simulink model "primary_node"  (Simulink 7.8)
settings: Solver=FixedStepDiscrete  SolverMode=SingleTasking  StartTime=0.0  StopTime=10.0  FixedStep=0.01  RelTol=1e-3
InitFcn:
  | clear all
  | missions
  | common
  | physical_constants
  | initial_values
  | l2plus
values from neighbouring files (symbols this model uses):
  InitialPoint = 0    [l2plus.m]
  IPStar = 0    [l2plus.m]
  lla_ltp_gain = [r * (pi / 180 / 1e7); v * cos(ref_lla(1)) * (pi / 180 / 1e7); 1e-6]    [common.m]
  MaxDwnPthStar = 1    [l2plus.m]
  ref_lla_sense = int32([36.963765 * 1e7; -122.00191 * 1e7; 0 * 1e6])    [common.m]
  switchDistance = 4    [l2plus.m]
  T_step = 0.01    [common.m]
  tanIntercept = tan( 45*pi/180 )    [l2plus.m]
  TStar = single(2)    [l2plus.m]
  Turn2Track = 0    [l2plus.m]
  wheelbase = 3.27    [physical_constants.m]
undefined symbols (not defined in the file or in its folder): ANmax, ClearGpsData, ClearRudderAngle, cpInitCommunications, DiscIntNeverNeededParam, GetGpsDataPacked, GetRcNodeAvailability, GetThrottleDataPacked, Init_onlyOnce, Init_Reset, MatlabGetMavLinkManualControl, MavLinkEvaluateMissionState, MavLinkEvaluateParameterState, MavLinkReceive, MavLinkScheduleCurrentMission, MavLinkScheduleGpsOrigin, MavLinkTransmit, NodeTransmitStatus, PrimaryNodeInit, RudderSendAngleCommand, SendThrottleCommand, test_waypoints, u1, u2, y1
libraries: dsPICdrivers x32, uSimLib x21, simulink x19, ecan_dspic x2, etargetslib x2, simulink_need_slupdate x1
(part 1 of 2)
CloseFcn:
  | rtwprivate ssgencode ModelCloseRequest code_gen
settings Model: Creator=bwmairs  LastModifiedBy=Bryant
settings OptimizationCC: BlockReduction=off  InlineParams=on  InlineInvariantSignals=on  PassReuseOutputArgsAs=Individual arguments  ZeroExternalMemoryAtStartup=off  ZeroInternalMemoryAtStartup=off  InitFltsAndDblsToZero=on  NoFixptDivByZeroProtection=on  EfficientFloat2IntCast=on  OptimizeModelRefInitCode=on
settings DebuggingCC: ReadBeforeWriteMsg=DisableAll  WriteAfterWriteMsg=DisableAll  WriteAfterReadMsg=DisableAll  UnderspecifiedInitializationDetection=Simplified  ParameterOverflowMsg=warning  FcnCallInpInsideContextMsg=Use local settings  UniqueDataStoreMsg=error
settings HardwareCC: ProdBitPerInt=16  ProdBitPerPointer=16  ProdIntDivRoundTo=Zero  ProdEndianess=LittleEndian  ProdWordSize=16  ProdHWDeviceType=16-bit Generic
settings ModelReferenceCC: ModelReferenceNumInstancesAllowed=Single
settings SFSimCC: SimParseCustomCode=off
settings RTWCC: SystemTargetFile=dspic.tlc  GenCodeOnly=on  MakeCommand=make_CreateMPLAB  TemplateMakefile=dspic_pic30_gcc.tmf  PostCodeGenCommand=dsPIC_Compile()  Description=Embedded Target for Microchip dsPIC (real-time)  ProcessScript=dspic_make_rtw_hook  RTWCompilerOptimization=On
settings RTWCC: CustomInclude=|
  | ../../../mavlink/C/include_v1.0/sealion
  | clib
  | ../Libs/C
settings RTWCC: CustomSource=|
  | clib/PrimaryNode.c
  | clib/EcanSensors.c
  | clib/MavlinkGlue.c
  | 
  | ../Libs/C/Acs300.c
  | ../Libs/C/MessageScheduler.c
  | ../Libs/C/Nmea2000.c
  | ../Libs/C/Nmea2000Encode.c
  | ../Libs/C/Rudder.c
  | ../Libs/C/Uart1.c
  | ../Libs/C/CanMessages.c
  | ../Libs/C/Traps.c
  | ../Libs/C/DEE.c
  | ../Libs/C/DEES.s
  | ../Libs/C/Node.c
  | ../Libs/C/CircularBuffer.c
  | 
  | ../../../ECAN_dspic/ecanFunctions.c
settings CodeAppCC: IgnoreCustomStorageClasses=off  IgnoreTestpoints=on
settings STFCustomTargetCC: TargetFunctionLibrary=C89/C90 (ANSI)  IncludeMdlTerminateFcn=off  GeneratePreprocessorConditionals=Use local settings  CombineOutputUpdateFcns=on  SuppressErrorStatus=on  ERTCustomFileBanners=on  SupportComplex=off  SupportContinuousTime=off  SupportNonInlinedSFcns=off  SystemTargetFile=dspic.tlc
settings ERTTargetCC: TargetFunctionLibrary=C89/C90 (ANSI)  MultiwordLength=2048  ParMdlRefBuildCompliant=off  CompOptLevelCompliant=off  ConcurrentExecutionCompliant=off  IncludeMdlTerminateFcn=off  SuppressErrorStatus=on  ERTFirstTimeCompliant=off  SupportComplex=off  ModelStepFunctionPrototypeControlCompliant=off  CPPClassGenCompliant=off  ExtModeMexFile=ext_serial_win32_comm  InlinedParameterPlacement=NonHierarchical  ERTSrcFileBannerTemplate=dsPIC_code_template.cgt  ERTHdrFileBannerTemplate=dsPIC_code_template.cgt  ERTDataSrcFileTemplate=dsPIC_code_template.cgt  ERTDataHdrFileTemplate=dsPIC_code_template.cgt  ERTCustomFileTemplate=dsPIC_main.tlc  SuppressUnreachableDefaultCases=off
settings CustomProperty: DataType=string  Value=C:\PROGRA~1\MATLAB\R2011b\bin\win64\gmake

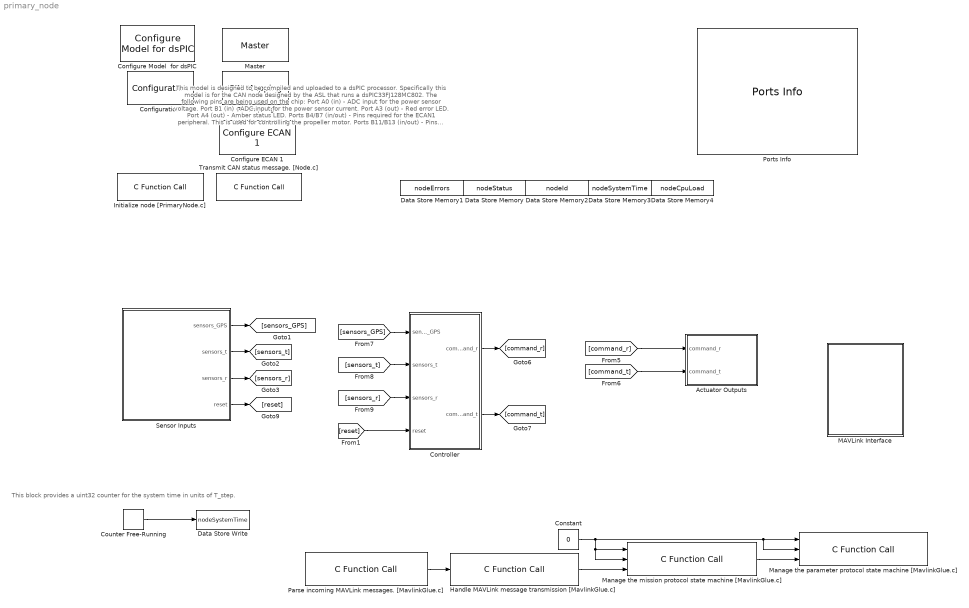
== system primary_node ==
  note: This model is designed to be compiled and uploaded to a dsPIC processor.
      | Specifically this model is for the CAN node designed by the ASL that runs a dsPIC33FJ128MC802.
      | The following pins are being used on the chip:
      | Port A0 (in) - ADC input for the power sensor voltage.
      | Port B1 (in) - ADC input for the power sensor current.
      | Port A3 (out) - Red error LED.
      | Port A4 (out) - Amber status LED.
      | Ports B4/B7 (in/out) - Pins required for the ECAN1 peripheral. This is used for controlling the propeller motor.
      | Ports B11/B13 (in/out) - Pins required for the UART1 peripheral used for groundstation communications.
      |
      | Switching between the autonomous controller and manual control involves using the landing gear channel. When
      | it's enabled, it's under autonomous control. This can only be changed when the RC transmitter is on and connected and
      | is never changed otherwise.
  note: This block provides a uint32 counter for the system time in units of T_step.
  Actuator Outputs : Subsystem
  Configuration : dsPICdrivers/Configuration  double64=on
  Configure ECAN 1 : ecan_dspic/Configure ECAN 1  frame_setting=on  mode=Normal  dma_rx_chan=2  dma_tx_chan=0  baud=250000  ps1=8  pd=5  ps2=6  sjw=4  tq=20  triple_sample=on  dma_buf_size=4 buffers  rx_bufs=[1]  tx_bufs=[0]  buf_0_tx_pri=Highest  buf_0_rte=No  buf_1_tx_pri=Highest  buf_1_rte=No  buf_2_tx_pri=Lowest  buf_2_rte=No  buf_3_tx_pri=Lowest  buf_3_rte=No  buf_4_tx_pri=Lowest  buf_4_rte=No  buf_5_tx_pri=Lowest  buf_5_rte=No  buf_6_tx_pri=Lowest  buf_6_rte=No  buf_7_tx_pri=Lowest  buf_7_rte=No  mask_0=0  mask_0_mide=Match std or ext  mask_1=0  mask_1_mide=Match std or ext  mask_2=0  mask_2_mide=Match std or ext  filters=[0]  filter_0=0  filter_0_mask=0  filter_0_exide=Match only standard  filter_0_buf=1  filter_1=hex2dec('401')  filter_1_mask=0  filter_1_exide=Match only standard  filter_1_buf=2  filter_2=hex2dec('402')  filter_2_mask=0  filter_2_exide=Match only standard  filter_2_buf=3  filter_3=0  filter_3_mask=0  filter_3_exide=Match only standard  filter_3_buf=0  filter_4=0  filter_4_mask=0  filter_4_exide=Match only standard  filter_4_buf=0  filter_5=0  filter_5_mask=0  filter_5_exide=Match only standard  filter_5_buf=0  filter_6=0  filter_6_mask=0  filter_6_exide=Match only standard  filter_6_buf=0  filter_7=0  filter_7_mask=0  filter_7_exide=Match only standard  filter_7_buf=0  filter_8=0  filter_8_mask=0  filter_8_exide=Match only standard  filter_8_buf=0  filter_9=0  filter_9_mask=<empty>  filter_9_exide=Match only standard  filter_9_buf=0  filter_10=0  filter_10_mask=0  filter_10_exide=Match only standard  filter_10_buf=0  filter_11=0  filter_11_mask=0  filter_11_exide=Match only standard  filter_11_buf=0  filter_12=0  filter_12_mask=0  filter_12_exide=Match only standard  filter_12_buf=0  filter_13=0  filter_13_mask=0  filter_13_exide=Match only standard  filter_13_buf=0  filter_14=0  filter_14_mask=0  filter_14_exide=Match only standard  filter_14_buf=0  filter_15=0  filter_15_mask=0  filter_15_exide=Match only standard  filter_15_buf=0
  Configure Model  for dsPIC : dsPICdrivers/Simulink Configuration/Configure Model  for dsPIC
  Constant : Constant  Value=0  OutDataTypeStr=uint8
  Controller : Subsystem
  Counter Free-Running : simulink/Sources/Counter Free-Running  NumBits=32  tsamp=T_step
  Data Store Memory : DataStoreMemory  DataStoreName=nodeStatus  ReadBeforeWriteMsg=warning  WriteAfterWriteMsg=warning  WriteAfterReadMsg=warning  OutDataTypeStr=uint16
      settings: RTWStateStorageClass=ImportedExtern
  Data Store Memory1 : DataStoreMemory  DataStoreName=nodeErrors  ReadBeforeWriteMsg=warning  WriteAfterWriteMsg=warning  WriteAfterReadMsg=warning  OutDataTypeStr=uint16
      settings: RTWStateStorageClass=ImportedExtern
  Data Store Memory2 : DataStoreMemory  DataStoreName=nodeId  ReadBeforeWriteMsg=warning  WriteAfterWriteMsg=warning  WriteAfterReadMsg=warning  OutDataTypeStr=uint8
      settings: RTWStateStorageClass=ImportedExtern
  Data Store Memory3 : DataStoreMemory  DataStoreName=nodeSystemTime  ReadBeforeWriteMsg=warning  WriteAfterWriteMsg=warning  WriteAfterReadMsg=warning  OutDataTypeStr=uint32
      settings: RTWStateStorageClass=ImportedExtern
  Data Store Memory4 : DataStoreMemory  DataStoreName=nodeCpuLoad  ReadBeforeWriteMsg=warning  WriteAfterWriteMsg=warning  WriteAfterReadMsg=warning  OutDataTypeStr=uint8
      settings: RTWStateStorageClass=ImportedExtern
  Data Store Write : DataStoreWrite  DataStoreName=nodeSystemTime
  Handle MAVLink message transmission [MavlinkGlue.c] : dsPICdrivers/OTHERS/C Function Call  Tag=dsPIC_dsPIC_CFunctionCall  FctUpdate=Output Function  fctName=MavLinkTransmit  INPUT_SIZE=1  INPUT1=--  INPUT2=--  INPUT3=--  OUTPUT_SIZE=1  OUTPUT1=--  SampleTime=.01  InputType=[ ]  OutputType=[ ]  FctDeclaration=extern void MavLinkTransmit();  FctCall=MavLinkTransmit();  OrderingInOutPopup=Input & Output  FctStart=None  FctStart_Name=Init_onlyOnce  FctStart_Declaration=inline extern void Init_onlyOnce();  FctStart_Call=Init_onlyOnce();  FctInit=None  FctInit_Name=Init_Reset  FctInit_Declaration=inline extern void Init_Reset();  FctInit_Call=Init_Reset();  PinDigitalInput=[]  PinDigitalOutput=[]  AnalogueInput=[]
  Initialize node [PrimaryNode.c] : dsPICdrivers/OTHERS/C Function Call  Tag=dsPIC_dsPIC_CFunctionCall  FctUpdate=None  fctName=cpInitCommunications  INPUT_SIZE=1  INPUT1=--  INPUT2=--  INPUT3=--  OUTPUT_SIZE=1  OUTPUT1=--  SampleTime=Inf  InputType=[]  OutputType=[]  FctDeclaration=extern void cpInitCommunications();  FctCall=cpInitCommunications();  OrderingInOutPopup=None  FctStart=Start Function (Call once and only once)  FctStart_Name=PrimaryNodeInit  FctStart_Declaration=inline extern void PrimaryNodeInit();  FctStart_Call=PrimaryNodeInit();  FctInit=None  FctInit_Name=Init_Reset  FctInit_Declaration=inline extern void Init_Reset();  FctInit_Call=Init_Reset();  PinDigitalInput=[]  PinDigitalOutput=[]  AnalogueInput=[]
  MAVLink Interface : Subsystem
  Manage the mission protocol state machine [MavlinkGlue.c] : dsPICdrivers/OTHERS/C Function Call  Tag=dsPIC_dsPIC_CFunctionCall  FctUpdate=Output Function  fctName=MavLinkEvaluateMissionState  INPUT_SIZE=1  INPUT1=uint8  INPUT2=uint8  INPUT3=--  OUTPUT_SIZE=1  OUTPUT1=--  SampleTime=.01  InputType=[ 2 2 ]  OutputType=[ ]  FctDeclaration=extern void MavLinkEvaluateMissionState(uint8_T u1, uint8_T u2);  FctCall=MavLinkEvaluateMissionState(%u1, %u2);  OrderingInOutPopup=Input & Output  FctStart=None  FctStart_Name=Init_onlyOnce  FctStart_Declaration=inline extern void Init_onlyOnce();  FctStart_Call=Init_onlyOnce();  FctInit=None  FctInit_Name=Init_Reset  FctInit_Declaration=inline extern void Init_Reset();  FctInit_Call=Init_Reset();  PinDigitalInput=[]  PinDigitalOutput=[]  AnalogueInput=[]
  Manage the parameter protocol state machine [MavlinkGlue.c] : dsPICdrivers/OTHERS/C Function Call  Tag=dsPIC_dsPIC_CFunctionCall  FctUpdate=Output Function  fctName=MavLinkEvaluateParameterState  INPUT_SIZE=1  INPUT1=uint8  INPUT2=uint8  INPUT3=--  OUTPUT_SIZE=1  OUTPUT1=--  SampleTime=.01  InputType=[ 2 2 ]  OutputType=[ ]  FctDeclaration=extern void MavLinkEvaluateParameterState(uint8_T u1, uint8_T u2);  FctCall=MavLinkEvaluateParameterState(%u1, %u2);  OrderingInOutPopup=Input  FctStart=None  FctStart_Name=Init_onlyOnce  FctStart_Declaration=inline extern void Init_onlyOnce();  FctStart_Call=Init_onlyOnce();  FctInit=None  FctInit_Name=Init_Reset  FctInit_Declaration=inline extern void Init_Reset();  FctInit_Call=Init_Reset();  PinDigitalInput=[]  PinDigitalOutput=[]  AnalogueInput=[]
  Master : dsPICdrivers/Master  Tag=dsPIC_MASTER  Priority=1  TimeStepType=Timer1  picType=33fj128MC802  fcy=40008571.4286  Quartz_33f=8e6  PLLActive_33f=on  fcyDesired_33f=40000000  tmr1="[8  50010  -0.00057131]"  tmr1Info="Time Step : 0.01  ;   Error : -0.00057131%  PR1=50010"  tmr2345="[0  0  0  0]"  tmr2345cfg=[-1 -1 -1 -1]  IOautoConf=on  typePort="[ 8   0   0  10  10   0   0   0   0   0   0   0   0   0   0   0   0   8   0   0  22   0   0  23   0   0   0  23  10  22   0  10   0   0   0   0   0   0   0   0   0   0   0   0   0   0   0   0   0   0   0   0   0   0   0   0   0   0   0   0   0   0   0   0   0   0   0   0   0   0   0   0   0   0   0   0   0   0   0   0   0   0   0   0   0   0   0   0   0   0   0   0   0   0   0   0   0   0   0   0   0   0   0   0   0   0   0   0   0   0   0   0 ]"  TRIS="[ 65511  26495  65535  65535  65535  65535  65535 ]"  ADPCFG=0  MasterBusyPort=None  MasterOverloadPort=None  FOSC=Internal Fast RC 7.37Mhz  ClockSwitchMonitor=Both disabled  TempProtection_33f=TEMP_ON  FPBOR=<empty>  PWRT=disable  MCLR=<empty>  ICD=ICS_PGD3  JTAGEN=JTAGEN_OFF  PowerSave=off  OverrideFcy=off  NewFcy=1e6  PR2345="[65535  65535  65535  65535]"
  PIN Mapping : dsPICdrivers/Peripheral MAPPING/PIN Mapping  Tag=dsPIC_PIN_Mapping  in_INT1=Not tied (VSS)  in_INT2=Not tied (VSS)  in_T2CK=Not tied (VSS)  in_T3CK=Not tied (VSS)  in_T4CK=Not tied (VSS)  in_T5CK=Not tied (VSS)  in_IC1=Not tied (VSS)  in_IC2=Not tied (VSS)  in_IC7=Not tied (VSS)  in_IC8=Not tied (VSS)  out_OC1=Not changed  out_OC2=Not changed  out_OC3=Not changed  out_OC4=Not changed  in_OCFA=Not tied (VSS)  in_FLTA1=Not tied (VSS)  in_FLTA2=Not tied (VSS)  in_QEA1=Not tied (VSS)  in_QEB1=Not tied (VSS)  in_INDX1=Not tied (VSS)  out_UPDN1=Not changed  out_UPDN2=Not changed  in_QEA2=Not tied (VSS)  in_QEB2=Not tied (VSS)  in_INDX2=Not tied (VSS)  in_U1RX=tied to RP13  out_U1TX=tied to RP11  in_U1CTS=Not tied (VSS)  out_U1RTS=Not changed  in_U2RX=Not tied (VSS)  out_U2TX=Not changed  in_U2CTS=Not tied (VSS)  out_U2RTS=Not changed  in_SDI1=Not tied (VSS)  out_SDO1=Not changed  in_SCK1=Not tied (VSS)  out_SCK1OUT=Not changed  in_SS1=Not tied (VSS)  out_SS1OUT=Not changed  in_SDI2=Not tied (VSS)  out_SDO2=Not changed  in_SCK2=Not tied (VSS)  out_SCK2OUT=Not changed  in_SS2=Not tied (VSS)  out_SS2OUT=Not changed  in_C1RX=tied to RP4  out_C1TX=tied to RP7  out_C1OUT=Not changed  out_C2OUT=Not changed
  Parse incoming MAVLink messages. [MavlinkGlue.c] : dsPICdrivers/OTHERS/C Function Call  Tag=dsPIC_dsPIC_CFunctionCall  FctUpdate=Output Function  fctName=MavLinkReceive  INPUT_SIZE=1  INPUT1=--  INPUT2=--  INPUT3=--  OUTPUT_SIZE=1  OUTPUT1=--  SampleTime=T_step  InputType=[ ]  OutputType=[ ]  FctDeclaration=extern void MavLinkReceive();  FctCall=MavLinkReceive();  OrderingInOutPopup=Output  FctStart=None  FctStart_Name=Init_onlyOnce  FctStart_Declaration=inline extern void Init_onlyOnce();  FctStart_Call=Init_onlyOnce();  FctInit=None  FctInit_Name=Init_Reset  FctInit_Declaration=inline extern void Init_Reset();  FctInit_Call=Init_Reset();  PinDigitalInput=[]  PinDigitalOutput=[]  AnalogueInput=[]
  Ports Info : dsPICdrivers/Ports Info  Tag=dsPIC_PortInfo
  Sensor Inputs : Subsystem
  Transmit CAN status message. [Node.c] : dsPICdrivers/OTHERS/C Function Call  Tag=dsPIC_dsPIC_CFunctionCall  FctUpdate=Output Function  fctName=NodeTransmitStatus  INPUT_SIZE=1  INPUT1=--  INPUT2=--  INPUT3=--  OUTPUT_SIZE=1  OUTPUT1=--  SampleTime=0.5  InputType=[ ]  OutputType=[ ]  FctDeclaration=extern void NodeTransmitStatus();  FctCall=NodeTransmitStatus();  OrderingInOutPopup=None  FctStart=None  FctStart_Name=NodeTransmitStatus  FctStart_Declaration=inline extern void NodeTransmitStatus();  FctStart_Call=NodeTransmitStatus();  FctInit=None  FctInit_Name=Init_Reset  FctInit_Declaration=inline extern void Init_Reset();  FctInit_Call=Init_Reset();  PinDigitalInput=[]  PinDigitalOutput=[]  AnalogueInput=[]
  wires:
  Sensor Inputs/1(sensors_GPS) -> [sensors_GPS]
  Sensor Inputs/2(sensors_t) -> [sensors_t]
  Sensor Inputs/3(sensors_r) -> [sensors_r]
  Controller/1(command_r) -> [command_r]
  Controller/2(command_t) -> [command_t]
  [sensors_GPS] -> Controller/1(sensors_GPS)
  [sensors_t] -> Controller/2(sensors_t)
  [sensors_r] -> Controller/3(sensors_r)
  [reset] -> Controller/4(reset)
  Sensor Inputs/4(reset) -> [reset]
  [command_r] -> Actuator Outputs/1(command_r)
  [command_t] -> Actuator Outputs/2(command_t)
  Counter Free-Running/1 -> Data Store Write/1
  Parse incoming MAVLink messages. [MavlinkGlue.c]/1 -> Handle MAVLink message transmission [MavlinkGlue.c]/1
  Handle MAVLink message transmission [MavlinkGlue.c]/1 -> Manage the mission protocol state machine [MavlinkGlue.c]/3
  Manage the mission protocol state machine [MavlinkGlue.c]/1 -> Manage the parameter protocol state machine [MavlinkGlue.c]/3
  Constant/1 -> Manage the mission protocol state machine [MavlinkGlue.c]/1, Manage the mission protocol state machine [MavlinkGlue.c]/2, Manage the parameter protocol state machine [MavlinkGlue.c]/1, Manage the parameter protocol state machine [MavlinkGlue.c]/2

== system primary_node/Actuator Outputs ==
  note: Propulsion is controlled here via a CAN interface to the motor driver board.
      | ECAN1 is used and several possible commands are transmitted: enable, disable,
      | or change speed, with speed being between -1023 and 1023 taken as a fraction
      | of total speed (1023).
  note: Rudder commands are controlled via a CAN interface to a CAN_node controller
      | at the stern of the vessel.
  command_r : Inport
  command_t : Inport  Port=2
  Detect Change : simulink/Logic and Bit Operations/Detect Change  vinit=0  InputProcessing=Inherited  OutDataTypeStr=uint8
  Detect Change1 : simulink/Logic and Bit Operations/Detect Change  vinit=0  InputProcessing=Inherited  OutDataTypeStr=uint8
  Transmit Angle Command : Subsystem  TreatAsAtomicUnit=on
  Transmit Throtle Command : Subsystem  TreatAsAtomicUnit=on
  wires:
  command_r/1 -> Detect Change/1, Transmit Angle Command/1(r_angle)
  command_t/1 -> Transmit Throtle Command/1(r_angle), Detect Change1/1
  Detect Change/1 -> Transmit Angle Command/Trigger
  Detect Change1/1 -> Transmit Throtle Command/Trigger

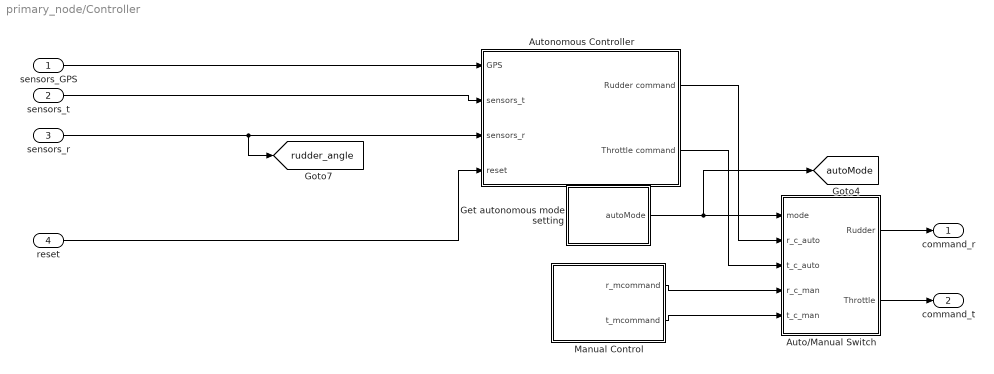
== system primary_node/Controller ==
  sensors_GPS : Inport
  sensors_t : Inport  Port=2
  sensors_r : Inport  Port=3
  reset : Inport  Port=4
  Auto/Manual Switch : Subsystem
  Autonomous Controller : Subsystem  Priority=1
  Get autonomous mode setting : Subsystem
  Manual Control : Subsystem
  command_r : Outport
  command_t : Outport  Port=2
  tag scope: autoMode=global, rudder_angle=global
  wires:
  sensors_t/1 -> Autonomous Controller/2(sensors_t)
  sensors_GPS/1 -> Autonomous Controller/1(GPS)
  Manual Control/1(r_mcommand) -> Auto/Manual Switch/4(r_c_man)
  Manual Control/2(t_mcommand) -> Auto/Manual Switch/5(t_c_man)
  reset/1 -> Autonomous Controller/4(reset)
  Autonomous Controller/1(Rudder command) -> Auto/Manual Switch/2(r_c_auto)
  Autonomous Controller/2(Throttle command) -> Auto/Manual Switch/3(t_c_auto)
  Auto/Manual Switch/1(Rudder) -> command_r/1
  Auto/Manual Switch/2(Throttle) -> command_t/1
  sensors_r/1 -> [rudder_angle], Autonomous Controller/3(sensors_r)
  Get autonomous mode setting/1(autoMode) -> Auto/Manual Switch/1(mode), [autoMode]

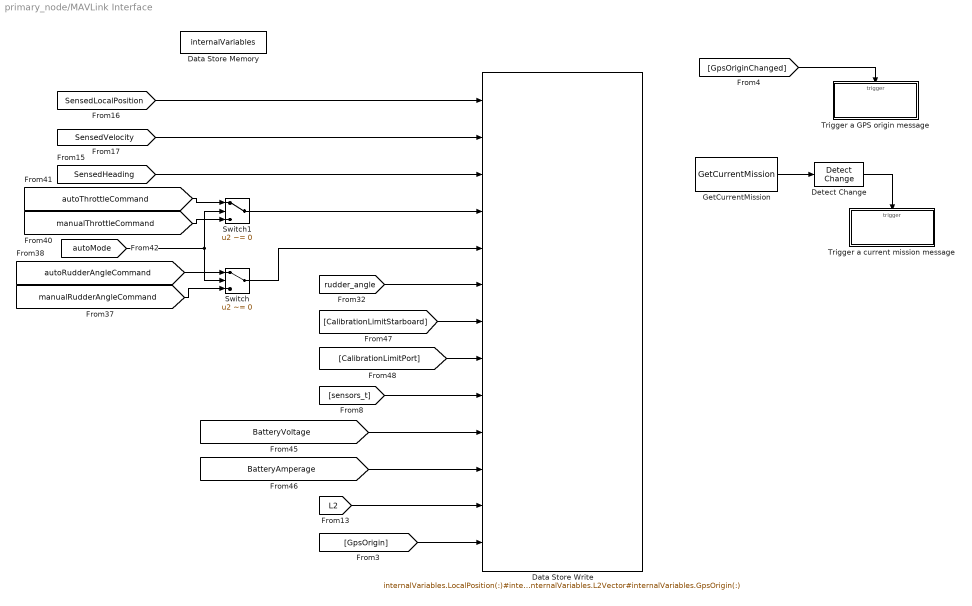
== system primary_node/MAVLink Interface ==
  Data Store Memory : DataStoreMemory  DataStoreName=internalVariables  OutDataTypeStr=Bus: MavlinkData
      settings: RTWStateStorageClass=ExportedGlobal
  Data Store Write : DataStoreWrite  DataStoreName=internalVariables  DataStoreElements=internalVariables.LocalPosition(:)#internalVariables.Velocity(:)#internalVariables.Heading#internalVariables.ThrottleCommand#internalVariables.RudderCommand#internalVariables.RudderPositionAngle#internalVariables.RudderCalLimitStarboard#internalVariables.RudderCalLimitPort#internalVariables.PropellerRpm#internalVariables.BatteryVoltage#internalVariables.BatteryAmperage#internalVariables.L2Vector#internalVariables.GpsOrigin(:)
  Detect Change : simulink/Logic and Bit Operations/Detect Change  vinit=0  InputProcessing=Inherited  OutDataTypeStr=boolean
  GetCurrentMission : uSimLib/Mission Manager/GetCurrentMission  sampleTime=T_step
  Switch : Switch  Criteria=u2 ~= 0
  Switch1 : Switch  Criteria=u2 ~= 0
  Trigger a GPS origin message : Subsystem  TreatAsAtomicUnit=on
  Trigger a current mission message : Subsystem  TreatAsAtomicUnit=on
  wires:
  [SensedLocalPosition] -> Data Store Write/1
  [SensedVelocity] -> Data Store Write/2
  [SensedHeading] -> Data Store Write/3
  [GpsOriginChanged] -> Trigger a GPS origin message/Trigger
  GetCurrentMission/1 -> Detect Change/1
  Detect Change/1 -> Trigger a current mission message/Trigger
  [autoMode] -> Switch1/2, Switch/2
  [autoThrottleCommand] -> Switch1/1
  [manualThrottleCommand] -> Switch1/3
  Switch1/1 -> Data Store Write/4
  [L2] -> Data Store Write/12
  [rudder_angle] -> Data Store Write/6
  [sensors_t] -> Data Store Write/9
  [autoRudderAngleCommand] -> Switch/1
  [manualRudderAngleCommand] -> Switch/3
  Switch/1 -> Data Store Write/5
  [BatteryVoltage] -> Data Store Write/10
  [BatteryAmperage] -> Data Store Write/11
  [CalibrationLimitStarboard] -> Data Store Write/7
  [CalibrationLimitPort] -> Data Store Write/8
  [GpsOrigin] -> Data Store Write/13

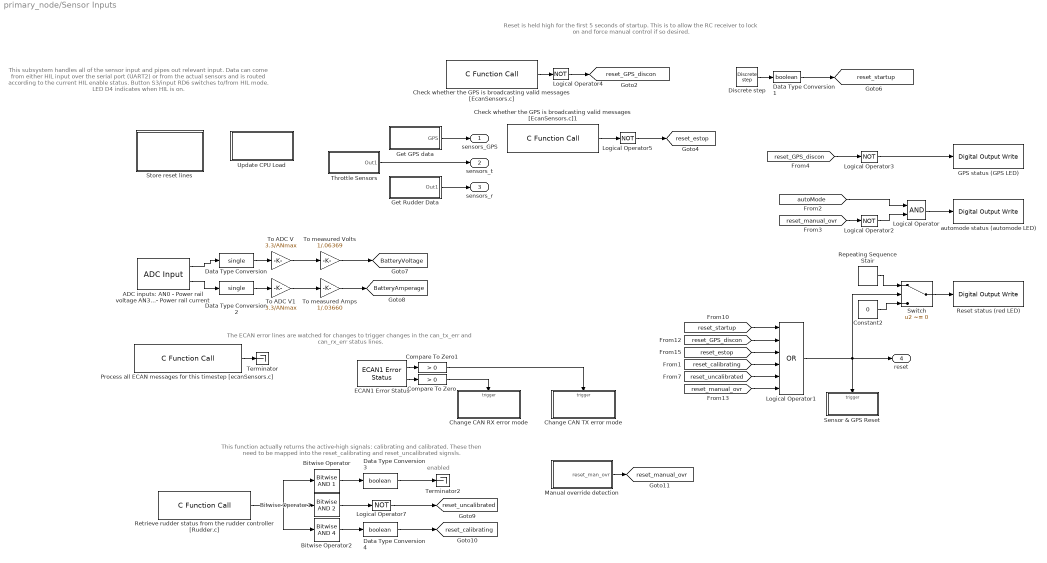
== system primary_node/Sensor Inputs ==
  note: This subsystem handles all of the sensor input and pipes out relevant input. Data can come
      | from either HIL input over the serial port (UART2) or from the actual sensors and is routed
      | according to the current HIL enable status. Button S3/input RD6 switches to/from HIL mode.
      | LED D4 indicates when HIL is on.
  note: Reset is held high for the first 5 seconds of startup. This is to allow
      | the RC receiver to lock on and force manual control if so desired.
  note: The ECAN error lines are watched for changes to trigger changes
      | in the can_tx_err and can_rx_err status lines.
  note: This function actually returns the active-high signals:
      | calibrating and calibrated. These then need to be
      | mapped into the reset_calibrating and reset_uncalibrated
      | signsls.
  note: enabled
  ADC inputs: AN0 - Power rail voltage AN3 - Power rail current : dsPICdrivers/Peripheral I//O/ADC Input  Tag=dsPIC_ADC  Priority=5  ADC_TYPE=12 bits  ADC_MODE=Continuous sampling & get last channel value  NbrSampleStep=1  VoltRefpopup="AVdd  -  AVss"  OutFormatBitspopup=0000 dddd dddd dddd : Integer  InterruptPriority=6  ANCHANNELS=[0 3]  MaxName=ANmax = 4095  Rin=0  ADCS=53  SAMC=1  Temperature=25  DMAChannel=7  SampleTime=T_step  Status="OK  |  Tsmp=6.749e-007 |  T/Channel=1.012e-005 |  Tall=2.025e-005"  SSRC=auto convert
  Bitwise Operator : simulink/Logic and Bit Operations/Bitwise Operator  logicop=AND  UseBitMask=on  BitMask=1  BitMaskRealWorld=Stored Integer
  Bitwise Operator1 : simulink/Logic and Bit Operations/Bitwise Operator  logicop=AND  UseBitMask=on  BitMask=2  BitMaskRealWorld=Stored Integer
  Bitwise Operator2 : simulink/Logic and Bit Operations/Bitwise Operator  logicop=AND  UseBitMask=on  BitMask=4  BitMaskRealWorld=Stored Integer
  Change CAN RX error mode : Subsystem  TreatAsAtomicUnit=on
  Change CAN TX error mode : Subsystem  TreatAsAtomicUnit=on
  Check whether the GPS is broadcasting valid messages [EcanSensors.c] : dsPICdrivers/OTHERS/C Function Call  Tag=dsPIC_dsPIC_CFunctionCall  FctUpdate=Output Function  fctName=GetGpsEnabled  INPUT_SIZE=1  INPUT1=--  INPUT2=--  INPUT3=--  OUTPUT_SIZE=1  OUTPUT1=uint8  SampleTime=T_step  InputType=[ ]  OutputType=[ 2 ]  FctDeclaration=extern uint8_T GetGpsEnabled();  FctCall=%y1 = GetGpsEnabled();  OrderingInOutPopup=None  FctStart=None  FctStart_Name=Init_onlyOnce  FctStart_Declaration=inline extern void Init_onlyOnce();  FctStart_Call=Init_onlyOnce();  FctInit=None  FctInit_Name=Init_Reset  FctInit_Declaration=inline extern void Init_Reset();  FctInit_Call=Init_Reset();  PinDigitalInput=[]  PinDigitalOutput=[]  AnalogueInput=[]
  Check whether the GPS is broadcasting valid messages [EcanSensors.c]1 : dsPICdrivers/OTHERS/C Function Call  Tag=dsPIC_dsPIC_CFunctionCall  FctUpdate=Output Function  fctName=GetPropActive  INPUT_SIZE=1  INPUT1=--  INPUT2=--  INPUT3=--  OUTPUT_SIZE=1  OUTPUT1=uint8  SampleTime=T_step  InputType=[ ]  OutputType=[ 2 ]  FctDeclaration=extern uint8_T GetPropActive();  FctCall=%y1 = GetPropActive();  OrderingInOutPopup=None  FctStart=None  FctStart_Name=Init_onlyOnce  FctStart_Declaration=inline extern void Init_onlyOnce();  FctStart_Call=Init_onlyOnce();  FctInit=None  FctInit_Name=Init_Reset  FctInit_Declaration=inline extern void Init_Reset();  FctInit_Call=Init_Reset();  PinDigitalInput=[]  PinDigitalOutput=[]  AnalogueInput=[]
  Compare To Zero : simulink/Logic and Bit Operations/Compare To Zero  relop=>  OutDataTypeStr=boolean
  Compare To Zero1 : simulink/Logic and Bit Operations/Compare To Zero  relop=>  OutDataTypeStr=boolean
  Constant2 : Constant  Value=0  OutDataTypeStr=boolean
  Data Type Conversion : DataTypeConversion  OutDataTypeStr=single
  Data Type Conversion1 : DataTypeConversion  OutDataTypeStr=boolean
  Data Type Conversion2 : DataTypeConversion  OutDataTypeStr=single
  Data Type Conversion3 : DataTypeConversion  OutDataTypeStr=boolean  RndMeth=Simplest
  Data Type Conversion4 : DataTypeConversion  OutDataTypeStr=boolean  RndMeth=Simplest
  Discrete step : uSimLib/Sources/Discrete step  start_value=1  end_value=0  transition_time=500
  ECAN1 Error Status : ecan_dspic/ECAN1 Error Status  ecan1_error_sample_time=T_step
  GPS status (GPS LED) : dsPICdrivers/Digital I//O/Digital Output Write  Tag=dsPIC_Digital_Output  Priority=5  PORT=B  Pin=[15]  Simultaneous=off  OrderingInOutPopup=None
  Get GPS data : Subsystem
  Get Rudder Data : Subsystem
  Logical Operator : Logic  AllPortsSameDT=off  OutDataTypeStr=boolean
  Logical Operator1 : Logic  Operator=OR  Inputs=6  AllPortsSameDT=off  OutDataTypeStr=boolean
  Logical Operator{2..5,7} (5 alike) : Logic  Operator=NOT  AllPortsSameDT=off  OutDataTypeStr=boolean
  Manual override detection : Subsystem
  Process all ECAN messages for this timestep [ecanSensors.c] : dsPICdrivers/OTHERS/C Function Call  Tag=dsPIC_dsPIC_CFunctionCall  FctUpdate=Output Function  fctName=ProcessAllEcanMessages  INPUT_SIZE=1  INPUT1=--  INPUT2=--  INPUT3=--  OUTPUT_SIZE=1  OUTPUT1=uint8  SampleTime=.01  InputType=[ ]  OutputType=[ 2 ]  FctDeclaration=extern uint8_T ProcessAllEcanMessages();  FctCall=%y1 = ProcessAllEcanMessages();  OrderingInOutPopup=None  FctStart=None  FctStart_Name=Init_onlyOnce  FctStart_Declaration=inline extern void Init_onlyOnce();  FctStart_Call=Init_onlyOnce();  FctInit=None  FctInit_Name=Init_Reset  FctInit_Declaration=inline extern void Init_Reset();  FctInit_Call=Init_Reset();  PinDigitalInput=[]  PinDigitalOutput=[]  AnalogueInput=[]
  Repeating Sequence Stair : simulink/Sources/Repeating Sequence Stair  OutValues=[1 0]  tsamp=.5  OutMin=[]  OutMax=[]  OutDataTypeStr=fixdt('boolean')  OutputDataTypeScalingMode=Specify via dialog  OutDataType=fixdt('boolean')  ConRadixGroup=Best Precision: Vector-wise  OutScaling=[]
  Reset status (red LED) : dsPICdrivers/Digital I//O/Digital Output Write  Tag=dsPIC_Digital_Output  Priority=5  PORT=A  Pin=[3]  Simultaneous=off  OrderingInOutPopup=None
  Retrieve rudder status from the rudder controller [Rudder.c] : dsPICdrivers/OTHERS/C Function Call  Tag=dsPIC_dsPIC_CFunctionCall  FctUpdate=Output Function  fctName=GetRudderStatus  INPUT_SIZE=1  INPUT1=--  INPUT2=--  INPUT3=--  OUTPUT_SIZE=1  OUTPUT1=uint8  SampleTime=T_step  InputType=[ ]  OutputType=[ 2 ]  FctDeclaration=extern uint8_T GetRudderStatus();  FctCall=%y1 = GetRudderStatus();  OrderingInOutPopup=None  FctStart=None  FctStart_Name=Init_onlyOnce  FctStart_Declaration=inline extern void Init_onlyOnce();  FctStart_Call=Init_onlyOnce();  FctInit=None  FctInit_Name=Init_Reset  FctInit_Declaration=inline extern void Init_Reset();  FctInit_Call=Init_Reset();  PinDigitalInput=[]  PinDigitalOutput=[]  AnalogueInput=[]
  Sensor & GPS Reset : Subsystem
  Store reset lines : Subsystem
      mask Display: disp('');
  Switch : Switch  Criteria=u2 ~= 0
  Terminator : Terminator
  Terminator2 : Terminator
  Throttle Sensors : Subsystem
  To ADC V : Gain  Gain=3.3/ANmax
  To ADC V1 : Gain  Gain=3.3/ANmax
  To measured Amps : Gain  Gain=1/.03660
  To measured Volts : Gain  Gain=1/.06369
  Update CPU Load : Subsystem
      mask Display: disp('');
  automode status (automode LED) : dsPICdrivers/Digital I//O/Digital Output Write  Tag=dsPIC_Digital_Output  Priority=5  PORT=B  Pin=[12]  Simultaneous=off  OrderingInOutPopup=None
  sensors_GPS : Outport
  sensors_t : Outport  Port=2
  sensors_r : Outport  Port=3
  reset : Outport  Port=4
  tag scope: BatteryAmperage=global, BatteryVoltage=global, reset_GPS_discon=global, reset_calibrating=global, reset_estop=global, reset_manual_ovr=global, reset_startup=global, reset_uncalibrated=global
  wires:
  Get Rudder Data/1(Out1) -> sensors_r/1
  Get GPS data/1(GPS) -> sensors_GPS/1
  Logical Operator1/1 -> reset/1, Sensor & GPS Reset/Trigger, Switch/2
  Discrete step/1 -> Data Type Conversion1/1
  Logical Operator4/1 -> [reset_GPS_discon]
  Data Type Conversion1/1 -> [reset_startup]
  Check whether the GPS is broadcasting valid messages [EcanSensors.c]1/1 -> Logical Operator5/1
  Process all ECAN messages for this timestep [ecanSensors.c]/1 -> Terminator/1
  ADC inputs: AN0 - Power rail voltage AN3 - Power rail current/2 -> Data Type Conversion2/1
  Throttle Sensors/1(Out1) -> sensors_t/1
  [reset_estop] -> Logical Operator1/3
  Compare To Zero/1 -> Change CAN RX error mode/Trigger
  Compare To Zero1/1 -> Change CAN TX error mode/Trigger
  To ADC V/1 -> To measured Volts/1
  To measured Volts/1 -> [BatteryVoltage]
  To ADC V1/1 -> To measured Amps/1
  To measured Amps/1 -> [BatteryAmperage]
  Data Type Conversion/1 -> To ADC V/1
  Data Type Conversion2/1 -> To ADC V1/1
  [reset_startup] -> Logical Operator1/1
  [reset_GPS_discon] -> Logical Operator1/2
  ADC inputs: AN0 - Power rail voltage AN3 - Power rail current/1 -> Data Type Conversion/1
  Data Type Conversion3/1 -> Terminator2/1
  Data Type Conversion4/1 -> [reset_calibrating]
  Retrieve rudder status from the rudder controller [Rudder.c]/1 -> Bitwise Operator/1, Bitwise Operator1/1, Bitwise Operator2/1
  Bitwise Operator/1 -> Data Type Conversion3/1
  Bitwise Operator1/1 -> Logical Operator7/1
  Bitwise Operator2/1 -> Data Type Conversion4/1
  Logical Operator7/1 -> [reset_uncalibrated]
  [reset_calibrating] -> Logical Operator1/4
  [reset_uncalibrated] -> Logical Operator1/5
  Switch/1 -> Reset status (red LED)/1
  Constant2/1 -> Switch/3
  Repeating Sequence Stair/1 -> Switch/1
  [reset_manual_ovr] -> Logical Operator1/6
  Manual override detection/1(reset_man_ovr) -> [reset_manual_ovr]
  [autoMode] -> Logical Operator/1
  [reset_manual_ovr] -> Logical Operator2/1
  Logical Operator2/1 -> Logical Operator/2
  [reset_GPS_discon] -> Logical Operator3/1
  Logical Operator3/1 -> GPS status (GPS LED)/1
  Logical Operator/1 -> automode status (automode LED)/1
  Check whether the GPS is broadcasting valid messages [EcanSensors.c]/1 -> Logical Operator4/1
  Logical Operator5/1 -> [reset_estop]
  ECAN1 Error Status/1 -> Compare To Zero1/1
  ECAN1 Error Status/2 -> Compare To Zero/1

== system primary_node/Actuator Outputs/Transmit Angle Command ==
  r_angle : Inport
  Trigger : TriggerPort
  Transmit rudder angle command [Rudder.c] : dsPICdrivers/OTHERS/C Function Call  Tag=dsPIC_dsPIC_CFunctionCall  FctUpdate=Output Function  fctName=RudderSendAngleCommand  INPUT_SIZE=1  INPUT1=real32  INPUT2=--  INPUT3=--  OUTPUT_SIZE=1  OUTPUT1=--  SampleTime=-1  InputType=[ 7 ]  OutputType=[ ]  FctDeclaration=extern void RudderSendAngleCommand(real32_T u1);  FctCall=RudderSendAngleCommand(%u1);  OrderingInOutPopup=None  FctStart=None  FctStart_Name=Init_onlyOnce  FctStart_Declaration=inline extern void Init_onlyOnce();  FctStart_Call=Init_onlyOnce();  FctInit=None  FctInit_Name=Init_Reset  FctInit_Declaration=inline extern void Init_Reset();  FctInit_Call=Init_Reset();  PinDigitalInput=[]  PinDigitalOutput=[]  AnalogueInput=[]
  wires:
  r_angle/1 -> Transmit rudder angle command [Rudder.c]/1

== system primary_node/Actuator Outputs/Transmit Throtle Command ==
  r_angle : Inport
  Trigger : TriggerPort
  Data Type Conversion : DataTypeConversion  OutDataTypeStr=int16  RndMeth=Simplest
  Transmit rudder angle command [Rudder.c] : dsPICdrivers/OTHERS/C Function Call  Tag=dsPIC_dsPIC_CFunctionCall  FctUpdate=Output Function  fctName=SendThrottleCommand  INPUT_SIZE=1  INPUT1=int16  INPUT2=--  INPUT3=--  OUTPUT_SIZE=1  OUTPUT1=--  SampleTime=-1  InputType=[ 3 ]  OutputType=[ ]  FctDeclaration=extern void SendThrottleCommand(int16_T u1);  FctCall=SendThrottleCommand(%u1);  OrderingInOutPopup=None  FctStart=None  FctStart_Name=Init_onlyOnce  FctStart_Declaration=inline extern void Init_onlyOnce();  FctStart_Call=Init_onlyOnce();  FctInit=None  FctInit_Name=Init_Reset  FctInit_Declaration=inline extern void Init_Reset();  FctInit_Call=Init_Reset();  PinDigitalInput=[]  PinDigitalOutput=[]  AnalogueInput=[]
  wires:
  r_angle/1 -> Data Type Conversion/1
  Data Type Conversion/1 -> Transmit rudder angle command [Rudder.c]/1

== system primary_node/Controller/Auto/Manual Switch ==
  note: This block handles switching between manual RC control and autonomous control.
      | Mode is a boolean that enables automatic control when true. Default is false.
  mode : Inport
  r_c_auto : Inport  Port=2
  t_c_auto : Inport  Port=3
  r_c_man : Inport  Port=4
  t_c_man : Inport  Port=5
  Switch : Switch  Criteria=u2 ~= 0
  Switch1 : Switch  Criteria=u2 ~= 0
  Rudder : Outport
  Throttle : Outport  Port=2
  wires:
  mode/1 -> Switch/2, Switch1/2
  r_c_auto/1 -> Switch/1
  r_c_man/1 -> Switch/3
  t_c_auto/1 -> Switch1/1
  t_c_man/1 -> Switch1/3
  Switch1/1 -> Throttle/1
  Switch/1 -> Rudder/1

== system primary_node/Controller/Autonomous Controller ==
  note: This subsystem currently provides autonomous control of the boat. It utilizes simple PID control
      | on the throttle and rudder based on desired location and bearing. Calculations are performed
      | to compute a straight-line path between current location and the programmed waypoint. The
      | boat then sets out to achieve this course.
  GPS : Inport
  sensors_t : Inport  Port=2
  sensors_r : Inport  Port=3
  reset : Inport  Port=4
  Discrete step : uSimLib/Sources/Discrete step  start_value=1  end_value=0  transition_time=1
  Initialize MissionList : Subsystem  TreatAsAtomicUnit=on
  Rudder Command : Subsystem
  State Keeper & Estimator : Subsystem
  Terminator1 : Terminator
  Throttle Command : Subsystem
  Rudder command : Outport
  Throttle command : Outport  Port=2
  wires:
  Discrete step/1 -> Initialize MissionList/Trigger
  reset/1 -> Rudder Command/2(Reset), Throttle Command/2(reset), State Keeper & Estimator/2(reset)
  State Keeper & Estimator/3(pos) -> Rudder Command/3(Local pos)
  State Keeper & Estimator/1(sensors_t) -> Throttle Command/1(sensors)
  State Keeper & Estimator/2(velocity) -> Rudder Command/1(Velocity)
  GPS/1 -> State Keeper & Estimator/3(gps)
  Throttle Command/1(command) -> Throttle command/1
  Rudder Command/1(Command) -> Rudder command/1
  sensors_r/1 -> Terminator1/1
  sensors_t/1 -> State Keeper & Estimator/1(throttle)

== system primary_node/Controller/Get autonomous mode setting ==
  Bitwise Operator : simulink/Logic and Bit Operations/Bitwise Operator  logicop=AND  UseBitMask=on  BitMask=hex2dec('1')  BitMaskRealWorld=Stored Integer
  Compare To Zero1 : simulink/Logic and Bit Operations/Compare To Zero  relop=~=  OutDataTypeStr=boolean
  Data Store Read : DataStoreRead  DataStoreName=nodeStatus
  autoMode : Outport
  wires:
  Data Store Read/1 -> Bitwise Operator/1
  Bitwise Operator/1 -> Compare To Zero1/1
  Compare To Zero1/1 -> autoMode/1

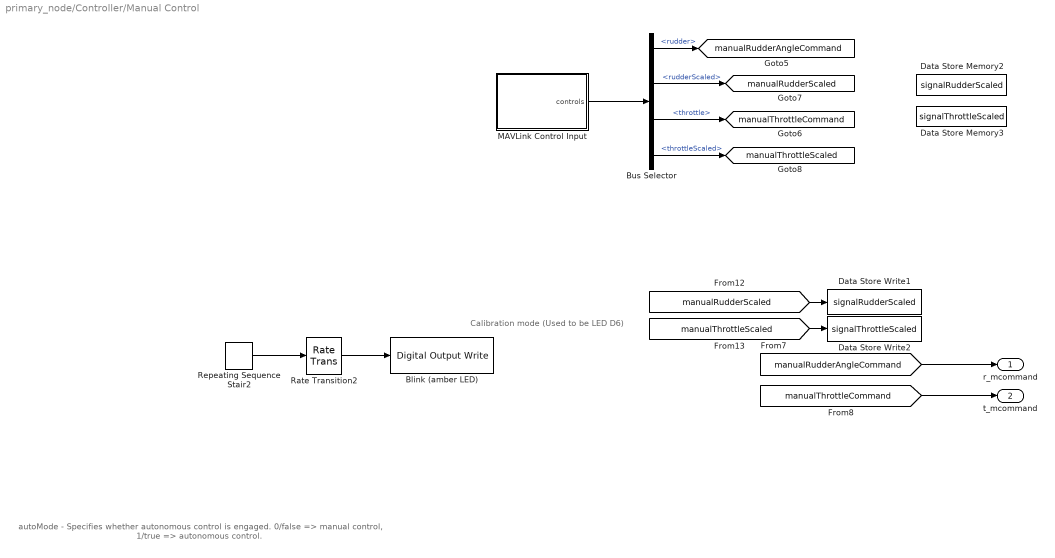
== system primary_node/Controller/Manual Control ==
  note: autoMode - Specifies whether autonomous control is engaged. 0/false => manual control, 1/true => autonomous control.
  note: Calibration mode
      | (Used to be LED D6)
  Blink (amber LED) : dsPICdrivers/Digital I//O/Digital Output Write  Tag=dsPIC_Digital_Output  Priority=5  PORT=A  Pin=[4]  Simultaneous=off  OrderingInOutPopup=None
  Bus Selector : BusSelector  OutputSignals=rudder,rudderScaled,throttle,throttleScaled
  Data Store Memory2 : DataStoreMemory  DataStoreName=signalRudderScaled  ReadBeforeWriteMsg=warning  WriteAfterWriteMsg=warning  WriteAfterReadMsg=warning  OutDataTypeStr=single
      settings: RTWStateStorageClass=ExportedGlobal
  Data Store Memory3 : DataStoreMemory  DataStoreName=signalThrottleScaled  ReadBeforeWriteMsg=warning  WriteAfterWriteMsg=warning  WriteAfterReadMsg=warning  OutDataTypeStr=single
      settings: RTWStateStorageClass=ExportedGlobal
  Data Store Write1 : DataStoreWrite  DataStoreName=signalRudderScaled
  Data Store Write2 : DataStoreWrite  DataStoreName=signalThrottleScaled
  MAVLink Control Input : Subsystem
  Rate Transition2 : RateTransition
  Repeating Sequence Stair2 : simulink/Sources/Repeating Sequence Stair  OutValues=[1 0]  tsamp=1  OutMin=[]  OutMax=[]  OutDataTypeStr=fixdt('boolean')  OutputDataTypeScalingMode=Specify via dialog  OutDataType=fixdt('boolean')  ConRadixGroup=Best Precision: Vector-wise  OutScaling=[]
  r_mcommand : Outport
  t_mcommand : Outport  Port=2
  tag scope: manualRudderAngleCommand=global, manualRudderScaled=global, manualThrottleCommand=global, manualThrottleScaled=global
  wires:
  Bus Selector/1 -> [manualRudderAngleCommand]  "<rudder>"
  Bus Selector/3 -> [manualThrottleCommand]  "<throttle>"
  Bus Selector/2 -> [manualRudderScaled]  "<rudderScaled>"
  Bus Selector/4 -> [manualThrottleScaled]  "<throttleScaled>"
  [manualRudderAngleCommand] -> r_mcommand/1
  [manualThrottleCommand] -> t_mcommand/1
  [manualThrottleScaled] -> Data Store Write2/1
  [manualRudderScaled] -> Data Store Write1/1
  MAVLink Control Input/1(controls) -> Bus Selector/1
  Repeating Sequence Stair2/1 -> Rate Transition2/1
  Rate Transition2/1 -> Blink (amber LED)/1

== system primary_node/MAVLink Interface/Trigger a GPS origin message ==
  Trigger : TriggerPort  PortDimensions=1
  Schedule GPS Origin message [MavlinkGlue.c] : dsPICdrivers/OTHERS/C Function Call  Tag=dsPIC_dsPIC_CFunctionCall  FctUpdate=Output Function  fctName=MavLinkScheduleGpsOrigin  INPUT_SIZE=1  INPUT1=--  INPUT2=--  INPUT3=--  OUTPUT_SIZE=1  OUTPUT1=--  SampleTime=-1  InputType=[ ]  OutputType=[ ]  FctDeclaration=extern void MavLinkScheduleGpsOrigin();  FctCall=MavLinkScheduleGpsOrigin();  OrderingInOutPopup=None  FctStart=None  FctStart_Name=Init_onlyOnce  FctStart_Declaration=inline extern void Init_onlyOnce();  FctStart_Call=Init_onlyOnce();  FctInit=None  FctInit_Name=Init_Reset  FctInit_Declaration=inline extern void Init_Reset();  FctInit_Call=Init_Reset();  PinDigitalInput=[]  PinDigitalOutput=[]  AnalogueInput=[]

== system primary_node/MAVLink Interface/Trigger a current mission message ==
  Trigger : TriggerPort
  Schedule a current mission message [MavlinkGlue.c] : dsPICdrivers/OTHERS/C Function Call  Tag=dsPIC_dsPIC_CFunctionCall  FctUpdate=Output Function  fctName=MavLinkScheduleCurrentMission  INPUT_SIZE=1  INPUT1=--  INPUT2=--  INPUT3=--  OUTPUT_SIZE=1  OUTPUT1=--  SampleTime=-1  InputType=[ ]  OutputType=[ ]  FctDeclaration=extern void MavLinkScheduleCurrentMission();  FctCall=MavLinkScheduleCurrentMission();  OrderingInOutPopup=None  FctStart=None  FctStart_Name=cpInitCommunications  FctStart_Declaration=inline extern void cpInitCommunications();  FctStart_Call=cpInitCommunications();  FctInit=None  FctInit_Name=Init_Reset  FctInit_Declaration=inline extern void Init_Reset();  FctInit_Call=Init_Reset();  PinDigitalInput=[]  PinDigitalOutput=[]  AnalogueInput=[]

== system primary_node/Sensor Inputs/Change CAN RX error mode ==
  Trigger : TriggerPort  TriggerType=either
  Bitwise Operator : simulink/Logic and Bit Operations/Bitwise Operator  logicop=XOR  UseBitMask=on  BitMask=hex2dec('40')  BitMaskRealWorld=Stored Integer
  Data Store Read : DataStoreRead  DataStoreName=nodeStatus
  Data Store Write : DataStoreWrite  DataStoreName=nodeStatus
  wires:
  Data Store Read/1 -> Bitwise Operator/1
  Bitwise Operator/1 -> Data Store Write/1

== system primary_node/Sensor Inputs/Change CAN TX error mode ==
  Trigger : TriggerPort  TriggerType=either
  Bitwise Operator1 : simulink/Logic and Bit Operations/Bitwise Operator  logicop=XOR  UseBitMask=on  BitMask=hex2dec('20')  BitMaskRealWorld=Stored Integer
  Data Store Read1 : DataStoreRead  DataStoreName=nodeStatus
  Data Store Write1 : DataStoreWrite  DataStoreName=nodeStatus
  wires:
  Data Store Read1/1 -> Bitwise Operator1/1
  Bitwise Operator1/1 -> Data Store Write1/1

== system primary_node/Sensor Inputs/Get GPS data ==
  Bus Creator : BusCreator  Inputs=6
  Byte Unpack : etargetslib/Byte Unpack  dimensions={[1],[1],[1],[1],[1],[1]}  datatypes={'int32', 'int32', 'int32', 'uint16', 'uint16', 'boolean'}  byteAlign=1
  Retrieve GPS data [ecanSensors.c] : dsPICdrivers/OTHERS/C Function Call  Tag=dsPIC_dsPIC_CFunctionCall  FctUpdate=Output Function  fctName=GetGpsDataPacked  INPUT_SIZE=1  INPUT1=--  INPUT2=--  INPUT3=--  OUTPUT_SIZE=17  OUTPUT1=uint8  SampleTime=T_step  InputType=[ ]  OutputType=[ 2 ]  FctDeclaration=extern void GetGpsDataPacked(uint8_T* y1);  FctCall=GetGpsDataPacked(*%y1);  OrderingInOutPopup=None  FctStart=None  FctStart_Name=Init_onlyOnce  FctStart_Declaration=inline extern void Init_onlyOnce();  FctStart_Call=Init_onlyOnce();  FctInit=None  FctInit_Name=Init_Reset  FctInit_Declaration=inline extern void Init_Reset();  FctInit_Call=Init_Reset();  PinDigitalInput=[]  PinDigitalOutput=[]  AnalogueInput=[]
  GPS : Outport
  wires:
  Byte Unpack/1 -> Bus Creator/1  "latitude"
  Byte Unpack/2 -> Bus Creator/2  "longitude"
  Byte Unpack/3 -> Bus Creator/3  "altitude"
  Bus Creator/1 -> GPS/1
  Byte Unpack/6 -> Bus Creator/6  "newData"
  Byte Unpack/4 -> Bus Creator/4  "cog"
  Byte Unpack/5 -> Bus Creator/5  "sog"
  Retrieve GPS data [ecanSensors.c]/1 -> Byte Unpack/1

== system primary_node/Sensor Inputs/Get Rudder Data ==
  note: Rudder data is stored within Rudder.c.
      | Data is fed in via CAN unless HIL is active,
      | in which case it's then received via UART.
  Retrieve rudder angle from the rudder controller [Rudder.c] : dsPICdrivers/OTHERS/C Function Call  Tag=dsPIC_dsPIC_CFunctionCall  FctUpdate=Output Function  fctName=GetRudderAngle  INPUT_SIZE=1  INPUT1=--  INPUT2=--  INPUT3=--  OUTPUT_SIZE=1  OUTPUT1=real32  SampleTime=.01  InputType=[ ]  OutputType=[ 7 ]  FctDeclaration=extern real32_T GetRudderAngle();  FctCall=%y1 = GetRudderAngle();  OrderingInOutPopup=None  FctStart=None  FctStart_Name=Init_onlyOnce  FctStart_Declaration=inline extern void Init_onlyOnce();  FctStart_Call=Init_onlyOnce();  FctInit=None  FctInit_Name=Init_Reset  FctInit_Declaration=inline extern void Init_Reset();  FctInit_Call=Init_Reset();  PinDigitalInput=[]  PinDigitalOutput=[]  AnalogueInput=[]
  Out1 : Outport
  wires:
  Retrieve rudder angle from the rudder controller [Rudder.c]/1 -> Out1/1

== system primary_node/Sensor Inputs/Manual override detection ==
  note: This block checks for status messages from the RC
      | control node. This relies on the sensor availability code
      | in `ecanSensors.c`. The RC Node is considered enabled
      | if it's broadcasting status messages. It's considered
      | active if it signifies that the RC transmitter is on, meaning
      | manual control is engaged.
      |
      | So the check done in this subsystem is to see if the RC
      | node is offline (!enabled) OR if it's online and active (active).
      | In either of these situations, the primary controller should
      | disable itself and let the RC node drive the vessel.
  Data Type Conversion : DataTypeConversion  OutDataTypeStr=boolean
  Demux : Demux  Outputs=2
  Get status info from the RC node [ecanSensors.c] : dsPICdrivers/OTHERS/C Function Call  Tag=dsPIC_dsPIC_CFunctionCall  FctUpdate=Output Function  fctName=GetRcNodeAvailability  INPUT_SIZE=1  INPUT1=--  INPUT2=--  INPUT3=--  OUTPUT_SIZE=2  OUTPUT1=uint8  SampleTime=T_step  InputType=[ ]  OutputType=[ 2 ]  FctDeclaration=extern void GetRcNodeAvailability(uint8_T* y1);  FctCall=GetRcNodeAvailability(*%y1);  OrderingInOutPopup=None  FctStart=None  FctStart_Name=Init_onlyOnce  FctStart_Declaration=inline extern void Init_onlyOnce();  FctStart_Call=Init_onlyOnce();  FctInit=None  FctInit_Name=Init_Reset  FctInit_Declaration=inline extern void Init_Reset();  FctInit_Call=Init_Reset();  PinDigitalInput=[]  PinDigitalOutput=[]  AnalogueInput=[]
  Logical Operator : Logic  Operator=OR  AllPortsSameDT=off  OutDataTypeStr=boolean
  Logical Operator2 : Logic  Operator=NOT  AllPortsSameDT=off  OutDataTypeStr=boolean
  reset_man_ovr : Outport
  wires:
  Get status info from the RC node [ecanSensors.c]/1 -> Data Type Conversion/1
  Logical Operator/1 -> reset_man_ovr/1
  Demux/1 -> Logical Operator2/1  "enabled"
  Demux/2 -> Logical Operator/2  "active"
  Data Type Conversion/1 -> Demux/1
  Logical Operator2/1 -> Logical Operator/1

== system primary_node/Sensor Inputs/Sensor & GPS Reset ==
  note: When the processor gets reset be sure to
      | also reset the various structs that persist data:
      | specifically the GPS and Sensor structs.
  Trigger : TriggerPort  TriggerType=either
  Clear GPS struct [EcanSensors.c] : dsPICdrivers/OTHERS/C Function Call  Tag=dsPIC_dsPIC_CFunctionCall  FctUpdate=Output Function  fctName=ClearGpsData  INPUT_SIZE=1  INPUT1=--  INPUT2=--  INPUT3=--  OUTPUT_SIZE=1  OUTPUT1=--  SampleTime=-1  InputType=[ ]  OutputType=[ ]  FctDeclaration=extern void ClearGpsData();  FctCall=ClearGpsData();  OrderingInOutPopup=None  FctStart=None  FctStart_Name=Init_onlyOnce  FctStart_Declaration=inline extern void Init_onlyOnce();  FctStart_Call=Init_onlyOnce();  FctInit=None  FctInit_Name=Init_Reset  FctInit_Declaration=inline extern void Init_Reset();  FctInit_Call=Init_Reset();  PinDigitalInput=[]  PinDigitalOutput=[]  AnalogueInput=[]
  Clear rudder data struct [Rudder.c] : dsPICdrivers/OTHERS/C Function Call  Tag=dsPIC_dsPIC_CFunctionCall  FctUpdate=Output Function  fctName=ClearRudderAngle  INPUT_SIZE=1  INPUT1=--  INPUT2=--  INPUT3=--  OUTPUT_SIZE=1  OUTPUT1=--  SampleTime=-1  InputType=[ ]  OutputType=[ ]  FctDeclaration=extern void ClearRudderAngle();  FctCall=ClearRudderAngle();  OrderingInOutPopup=None  FctStart=None  FctStart_Name=Init_onlyOnce  FctStart_Declaration=inline extern void Init_onlyOnce();  FctStart_Call=Init_onlyOnce();  FctInit=None  FctInit_Name=Init_Reset  FctInit_Declaration=inline extern void Init_Reset();  FctInit_Call=Init_Reset();  PinDigitalInput=[]  PinDigitalOutput=[]  AnalogueInput=[]

== system primary_node/Sensor Inputs/Store reset lines ==
  Bitwise-combine : Subsystem
  Constant : Constant  Value=false  OutDataTypeStr=boolean
  Constant1 : Constant  Value=false  OutDataTypeStr=boolean
  Data Store Write : DataStoreWrite  DataStoreName=nodeErrors
  Data Type Conversion3 : DataTypeConversion  OutDataTypeStr=uint16
  wires:
  [reset_startup] -> Bitwise-combine/1(bit0)
  [reset_GPS_discon] -> Bitwise-combine/4(bit3)
  Constant/1 -> Bitwise-combine/2(bit1)
  [reset_calibrating] -> Bitwise-combine/6(bit5)
  [reset_uncalibrated] -> Bitwise-combine/7(bit6)
  [reset_estop] -> Bitwise-combine/8(bit7)
  Bitwise-combine/1(Out1) -> Data Type Conversion3/1  "reset"
  Data Type Conversion3/1 -> Data Store Write/1
  [reset_manual_ovr] -> Bitwise-combine/5(bit4)
  Constant1/1 -> Bitwise-combine/3(bit2)

== system primary_node/Sensor Inputs/Throttle Sensors ==
  note: If a status message hasn't been received for 2.1 seconds, a reset
      | signal is activated. The status messages for the ACS300 are not
      | sent when it is in reset, so this will catch when the estop is active.
      |
      | This also serves to check that the CAN hardware is working correctly,
      | which I have had trouble with in the past.
  Retrieve throttle data from the ACS300 [ecanSensors.c] : dsPICdrivers/OTHERS/C Function Call  Tag=dsPIC_dsPIC_CFunctionCall  FctUpdate=Output Function  fctName=GetThrottleDataPacked  INPUT_SIZE=1  INPUT1=--  INPUT2=--  INPUT3=--  OUTPUT_SIZE=3  OUTPUT1=uint8  SampleTime=.01  InputType=[ ]  OutputType=[ 2 ]  FctDeclaration=extern void GetThrottleDataPacked(uint8_T* y1);  FctCall=GetThrottleDataPacked(*%y1);  OrderingInOutPopup=None  FctStart=None  FctStart_Name=Init_onlyOnce  FctStart_Declaration=inline extern void Init_onlyOnce();  FctStart_Call=Init_onlyOnce();  FctInit=None  FctInit_Name=Init_Reset  FctInit_Declaration=inline extern void Init_Reset();  FctInit_Call=Init_Reset();  PinDigitalInput=[]  PinDigitalOutput=[]  AnalogueInput=[]
  Terminator1 : Terminator
  Unpack throttle data : MATLAB Function  TreatAsAtomicUnit=on
  Out1 : Outport
  wires:
  Retrieve throttle data from the ACS300 [ecanSensors.c]/1 -> Unpack throttle data/1(u)
  Unpack throttle data/1(throttle) -> Out1/1
  Unpack throttle data/2(newData) -> Terminator1/1
